simulink library "uavsimblockset"  (Simulink 8.6)
settings: Solver=ode45  StartTime=0.0  StopTime=10.0  RelTol=1e-3
undefined symbols (not defined in the file or in its folder): aircraftmask_displayVortices, aircraftmask_ID, DiscIntNeverNeededParam, uavsim
undefined symbols (not defined in the file): aircraftmask_originNED_ECEF_rrm, aircraftmask_p0_NED_m, aircraftmask_phithetapsi0, aircraftmask_pqr0, aircraftmask_uvw0, fflib_degdegm2rrm, flat2lla
libraries: uavsimBlockset_ServoHS55 x5, aerolibtransform2 x4, aerolibutil x3, uavsimBlockset_UAV3DInterface x3, uavsimblockset_SixDOFKinematics x2, simulink_extras x2, uavsimBlockset_Cularis_withUAV3D x2, uavsimBlockset_ElectricPropulsion x2, formationFlyingBlockset x2, uavsimBlockset_DerivedAerodynamicConditions x2, uavsimBlockset_alphabetaVa2uvw x1, uavsimBlockset_AirspeedController x1
(part 1 of 2)
settings Model: Creator=mstolle  LastModifiedBy=j.bolting

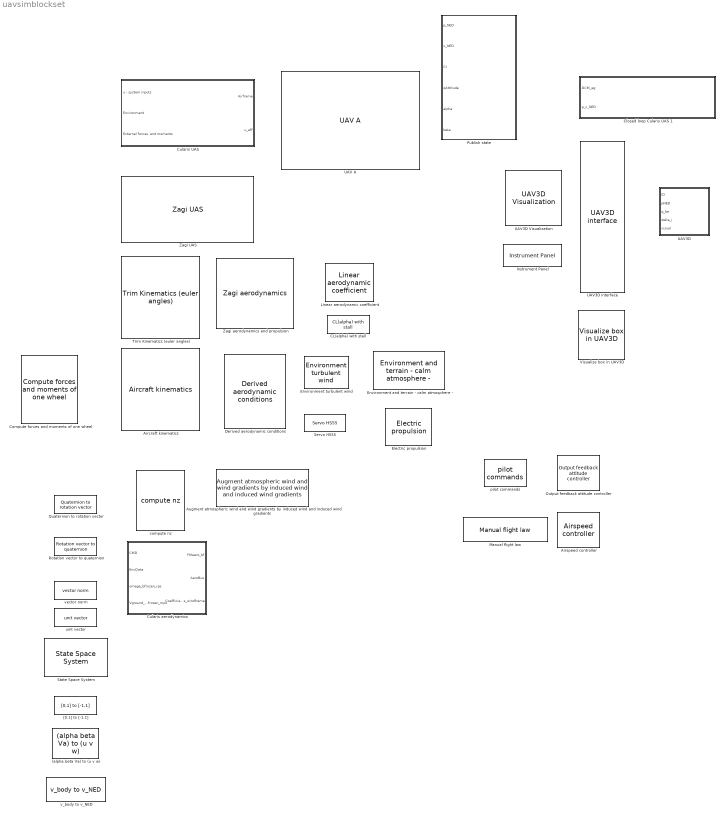
== system uavsimblockset ==
  (alpha beta Va) to (u v w) : uavsimBlockset_alphabetaVa2uvw/(alpha beta Va) to (u v w)
  Aircraft kinematics : uavsimblockset_SixDOFKinematics/Aircraft kinematics  mask_inertia="[ 0.98244, 0, -0.1204; 0,1.135,  0; -0.1204, 0,1.759]"  mask_mass=13.5  mask_P0_ECEF_rrm=mask_zagi_p0_ECEF_lla  mask_originNED_ECEF_rrm=0  mask_uvw0=mask_aerosonde_uvw0  mask_phithetapsi0=mask_aerosonde_phithetapsi0  mask_omega0=mask_aerosonde_pqr0
  Airspeed controller : uavsimBlockset_AirspeedController/Airspeed controller  mask_K=0
  Augment atmospheric wind and wind gradients by induced wind and induced wind gradients : uavsimBlockset_AugmentWind/Augment atmospheric wind and wind gradients by induced wind and induced wind gradients
  CL(alpha) with stall : uavsimBlockset_LiftCoefficientWithStall/CL(alpha) with stall  mask_M=0  mask_alpha0=0  mask_CL_0=0  mask_CL_alpha=0
  Closed loop Cularis UAS 1 : Subsystem  mask{closedloopmask_ID=2}
      mask prompts: closedloopmask_ID "UAS ID"
  Compute forces and moments of one wheel : uavsimBlockset_landinggear_onwheel/Compute forces and moments of one wheel
  Cularis UAS : Subsystem  mask{mask_cularis_phithetapsi0=aircraftmask_phithetapsi0, mask_cularis_p0_ECEF_lla=fflib_degdegm2rrm(flat2lla(aircraftmask_p0_NED_m, rad2deg(aircraftmask_originNED_ECEF_rrm(1:2)), 0, aircraftmask_originNED_ECEF_rrm(3))), mask_cularis_originNED_ECEF_rrm=aircraftmask_originNED_ECEF_rrm, mask_cularis_pqr0=aircraftmask_pqr0, mask_cularis_uvw0=aircraftmask_uvw0, uavsim=uavsim}
      mask prompts: mask_cularis_phithetapsi0 "Initial euler angles [rad]"; mask_cularis_p0_ECEF_lla "Initial position ECEF [rad rad m]"; mask_cularis_originNED_ECEF_rrm "Origin NED frame, ECEF-WGS84, [rad rad m]"; mask_cularis_pqr0 "Initial body rotation rates [rad/s]"; mask_cularis_uvw0 "Initial velocity body frame [m/s]"; uavsim "Parameter set"
      mask Display: image(imread('images/cularis.png'),[.3, .3, .4, .4])
  Cularis aerodynamics : Subsystem  AncestorBlock=uavsimBlockset_Cularis_Aerandpropulsion/Cularis aerodynamics and propulsion
  Derived aerodynamic conditions : uavsimBlockset_DerivedAerodynamicConditions/Derived aerodynamic conditions
  Electric propulsion : uavsimBlockset_ElectricPropulsion/Electric propulsion  mask_C_prop=0  mask_S_prop=0  mask_k_motor=0
  Environment turbulent wind : uavsimBlockset_Environment_turbulentWind/Environment turbulent wind  mask_constantwind_NED_mps=[0 0 0]'  mask_wingspan=1  mask_windON=mask_windON  mask_turbulenceON=1
  Environment and terrain - calm atmosphere - : uavsimBlockset_Environment_calmAtmosphere/Environment and terrain - calm atmosphere -  SystemSampleTime=-1
  Instrument Panel : uavsimBlockset_InstrumentPanel/Instrument Panel
  Linear aerodynamic coefficient : uavsimBlockset_LinearAerodynamicCoefficient/Linear aerodynamic coefficient  mask_C_0=0  mask_C_alpha=0  mask_C_beta=0  mask_C_alphaDot=0  mask_C_betaDot=0  mask_C_p=0  mask_C_q=0  mask_C_r=0  mask_C_delta_a=0  mask_C_delta_e=0  mask_C_delta_r=0  mask_C_delta_f=0  mask_C_Mach=0
  Manual flight law : uavsimBlockset_ManualLaw/Manual flight law  mask_scale_da=0  mask_scale_de=0  mask_scale_dr=0  mask_scale_den=0  mask_scale_df=0  mask_utrim=0
  Output feedback attitude controller : uavsimBlockset_quaternionAttitudeController/Output feedback attitude controller  mask_K=uavsim.control.linear.K_attitude
  Publish state : Subsystem  mask{mask_ID=aircraftmask_ID}
      mask prompts: mask_ID "ID"
  Quaternion to rotation vector : uavsimBlockset_Quaternion2Rotationvector/Quaternion to rotation vector
  Rotation vector to quaternion : uavsimBlockset_RotationVector2Quaternion/Rotation vector to quaternion
  Servo HS55 : uavsimBlockset_ServoHS55/Servo HS55  deflectionLimits_rad=[deg2rad(-45) deg2rad(45)]  rateLimit_enabled=on  outputLimit_enabled=on  mask_initialPosition=0
  State Space System : uavsimBlockset_StateSpaceSystem/State Space System  mask_a=0  mask_b=0  mask_c=0  mask_d=0  mask_x0=0
  Trim Kinematics (euler angles) : uavsimblockset_TrimKinematics/Trim Kinematics (euler angles)  mask_inertia=0  mask_mass=0  mask_P0_ECEF_m=0  mask_uvw0=0  mask_phithetapsi0=0  mask_omega0=0
  UAV A : uavsimBlockset_Cularis_withUAV3D/UAV A  aircraftmask_phithetapsi0=[uavsim.cularis.phithetapsi0(1:2); deg2rad(-30)]'  aircraftmask_p0_NED_m=[0 0 -50]  aircraftmask_originNED_ECEF_rrm=uavsim.originNED_ECEF_radradm  aircraftmask_pqr0=uavsim.cularis.omega0  aircraftmask_uvw0=uavsim.cularis.uvw0  aircraftmask_phithetapsi_trim=uavsim.cularis.phithetapsi0  aircraftmask_ID=1  aircraftmask_wakevortexenabled=off  aircraftmask_navigationLaw=4  uavsim=uavsim  leaderID=0  aircraftmask_displayUAV3D=on  aircraftmask_displayVortices=off
  UAV3D : Subsystem
  UAV3D Visualization : uavsimBlockset_UAV3DVisualization/UAV3D Visualization  mask_visual=0
  UAV3D interface : uavsimBlockset_UAV3DInterface/UAV3D interface  ip='localhost'  udpport=4445
  Visualize box in UAV3D : uavsimBlockset_UAV3D_visualizeBox/Visualize box in UAV3D
  Zagi UAS : uavsimBlockset_ZagiUAS/Zagi UAS  mask_zagi_phithetapsi0=[0 0 0]'  mask_zagi_p0_ECEF_lla=[0 0 50]'  mask_zagi_originNED_ECEF_rrm=0  mask_zagi_pqr0=[0 0 0]'  mask_zagi_uvw0=[30 0 0]  uavsim=uavsim
  Zagi aerodynamics and propulsion : uavsimBlockset_Zagi_Aerandpropulsion/Zagi aerodynamics
  "[0,1] to [-1,1]" : uavsimBlockset_01to11/[0,1] to [-1,1]
  compute nz : uavsimBlockset_ComputeNz/compute nz
  pilot commands : uavsimblockset_PilotCommands/pilot commands
  unit vector : uavsimBlockset_UnitVector/unit vector
  v_body to v_NED : uavsimblockset_vbody2vNED/v_body to v_NED
  vector norm : uavsimBlockset_VectorNorm/vector norm

== system uavsimblockset/Closed loop Cularis UAS 1 ==
  DCM_eg : Inport
  p_c_NED : Inport  Port=2
  Controllers : Subsystem
  UAV : uavsimBlockset_Cularis_withUAV3D/UAV A  aircraftmask_phithetapsi0=uavsim.formation(closedloopmask_ID).phithetapsi0  aircraftmask_p0_NED_m=uavsim.formation(closedloopmask_ID).p0_NED'  aircraftmask_originNED_ECEF_rrm=uavsim.originNED_ECEF_radradm  aircraftmask_pqr0=uavsim.formation(closedloopmask_ID).omega0  aircraftmask_uvw0=uavsim.formation(closedloopmask_ID).uvw0  aircraftmask_phithetapsi_trim=uavsim.formation(closedloopmask_ID).phithetapsi0  aircraftmask_ID=closedloopmask_ID  aircraftmask_wakevortexenabled=off  aircraftmask_navigationLaw=-1  uavsim=uavsim  leaderID=0  aircraftmask_displayUAV3D=on  aircraftmask_displayVortices=off
  wires:
  Controllers/1(u) -> UAV/1  "u_c"
  p_c_NED/1 -> Controllers/4(p_c_NED)
  DCM_eg/1 -> Controllers/3(DCM_eg)
  UAV/2 -> Controllers/2(id)
  UAV/1 -> Controllers/1(AirframeBus)

== system uavsimblockset/Cularis UAS ==
  u - system inputs : Inport  OutDataTypeStr=Bus: CMD
  Environment : Inport  Port=2  OutDataTypeStr=Bus: Environment
  External forces  and moments : Inport  Port=3
  Actuator dynamics neglected? : ManualSwitch  CurrentSetting=0
  Cularis actuators - time behaviour : Subsystem  TreatAsAtomicUnit=on
  ID2 : Constant  Value=aircraftmask_displayVortices
  Nonlinear aircraft model : Subsystem
  Publish state : Subsystem  TreatAsAtomicUnit=on
  Terminator1 : Terminator
  Wake vortex effects : formationFlyingBlockset/Wake vortex effects
  Airframe : Outport  OutDataTypeStr=Bus: Airframe
  u_eff : Outport  Port=2  OutDataTypeStr=Bus: CMD
  wires:
  u - system inputs/1 -> Cularis actuators - time behaviour/1(computed inputs), Actuator dynamics neglected?/2
  Cularis actuators - time behaviour/1(Effective  plant inputs) -> Actuator dynamics neglected?/1
  ID2/1 -> Wake vortex effects/4
  Publish state/2(Ci_w_out) -> Wake vortex effects/3
  Publish state/1(AiframeBus_out) -> Wake vortex effects/1
  Wake vortex effects/1 -> Nonlinear aircraft model/2(EnvData)
  Environment/1 -> Wake vortex effects/2
  Nonlinear aircraft model/3(FMprop) -> Terminator1/1
  Nonlinear aircraft model/2(Cwind) -> Publish state/2(Ci_w)
  Nonlinear aircraft model/1(Airframe) -> Airframe/1, Publish state/1(AirframeBus)
  Actuator dynamics neglected?/1 -> u_eff/1, Nonlinear aircraft model/1(CMD)
  External forces  and moments/1 -> Nonlinear aircraft model/3(FM_external)

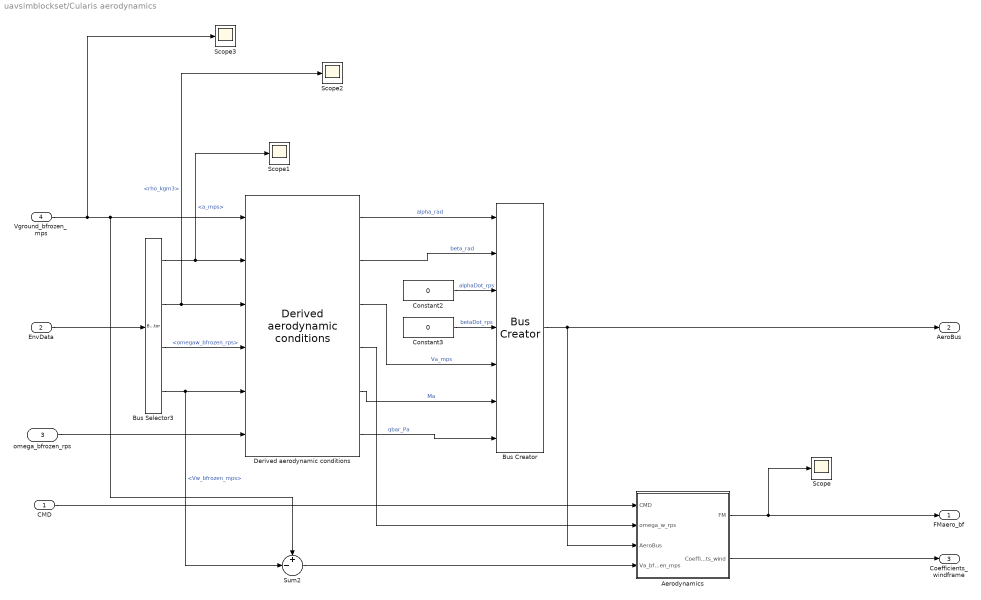
== system uavsimblockset/Cularis aerodynamics ==
  CMD : Inport  OutDataTypeStr=Bus: CMD
  EnvData : Inport  Port=2  OutDataTypeStr=Bus: Environment
  omega_bfrozen_rps : Inport  Port=3
  Vground_bfrozen_mps : Inport  Port=4
  Aerodynamics : Subsystem
  Bus Selector3 : BusSelector  OutputSignals=a_mps,rho_kgm3,omegaw_bfrozen_rps,Vw_bfrozen_mps
  Bus Creator : BusCreator  Inputs=7
  Constant2 : Constant  Value=0
  Constant3 : Constant  Value=0
  Derived aerodynamic conditions : uavsimBlockset_DerivedAerodynamicConditions/Derived aerodynamic conditions
  Scope{,1..3} (4 alike) : Scope
  Sum2 : Sum  Inputs=+-|  SaturateOnIntegerOverflow=on  InputSameDT=on  OutDataTypeStr=Inherit: Same as first input
  FMaero_bf : Outport
  AeroBus : Outport  Port=2  OutDataTypeStr=Bus: Aero
  Coefficients_windframe : Outport  Port=3
  wires:
  EnvData/1 -> Bus Selector3/1
  omega_bfrozen_rps/1 -> Derived aerodynamic conditions/6
  Aerodynamics/1(FM) -> FMaero_bf/1, Scope/1
  CMD/1 -> Aerodynamics/1(CMD)
  Aerodynamics/2(Coefficients_wind) -> Coefficients_windframe/1
  Bus Selector3/1 -> Derived aerodynamic conditions/2, Scope1/1  "<a_mps>"
  Bus Selector3/2 -> Derived aerodynamic conditions/3, Scope2/1  "<rho_kgm3>"
  Bus Selector3/3 -> Derived aerodynamic conditions/4  "<omegaw_bfrozen_rps>"
  Bus Selector3/4 -> Derived aerodynamic conditions/5, Sum2/2  "<Vw_bfrozen_mps>"
  Constant2/1 -> Bus Creator/3  "alphaDot_rps"
  Constant3/1 -> Bus Creator/4  "betaDot_rps"
  Vground_bfrozen_mps/1 -> Sum2/1, Derived aerodynamic conditions/1, Scope3/1
  Derived aerodynamic conditions/1 -> Bus Creator/1  "alpha_rad"
  Derived aerodynamic conditions/2 -> Bus Creator/2  "beta_rad"
  Derived aerodynamic conditions/3 -> Bus Creator/5  "Va_mps"
  Derived aerodynamic conditions/5 -> Bus Creator/6  "Ma"
  Derived aerodynamic conditions/6 -> Bus Creator/7  "qbar_Pa"
  Bus Creator/1 -> AeroBus/1, Aerodynamics/3(AeroBus)
  Sum2/1 -> Aerodynamics/4(Va_bfrozen_mps)
  Derived aerodynamic conditions/4 -> Aerodynamics/2(omega_w_rps)

== system uavsimblockset/Publish state ==
  p_NED : Inport
  v_NED : Inport  Port=2
  Cl : Inport  Port=3
  qAttitude : Inport  Port=4
  alpha : Inport  Port=5
  beta : Inport  Port=6
  Cularis vortex geometry parameters : formationFlyingBlockset/Cularis vortex geometry parameters  mask_ID=mask_ID
  Digital Clock : DigitalClock
  MATLAB Function1 : MATLAB Function  TreatAsAtomicUnit=on
  wires:
  Digital Clock/1 -> MATLAB Function1/8(tsim)
  Cularis vortex geometry parameters/1 -> MATLAB Function1/7(p)
  p_NED/1 -> MATLAB Function1/1(pNED)
  v_NED/1 -> MATLAB Function1/2(vNED)
  Cl/1 -> MATLAB Function1/3(CL)
  qAttitude/1 -> MATLAB Function1/4(qAttitude)
  alpha/1 -> MATLAB Function1/5(alpha)
  beta/1 -> MATLAB Function1/6(beta)

== system uavsimblockset/UAV3D ==
  ID : Inport
  pNED : Inport  Port=2
  q_be : Inport  Port=3
  delta_i : Inport  Port=4
  visual : Inport  Port=5
  Constant : Constant
  Demux : Demux  Outputs=5
  Demux1 : Demux
  Demux2 : Demux  Outputs=3
  UAV3D interface : uavsimBlockset_UAV3DInterface/UAV3D interface  ip='localhost'  udpport=4445
  wires:
  visual/1 -> UAV3D interface/14
  delta_i/1 -> Demux/1
  Demux/5 -> UAV3D interface/13
  Demux/4 -> UAV3D interface/12
  Demux/3 -> UAV3D interface/11
  Demux/2 -> UAV3D interface/10
  Demux/1 -> UAV3D interface/9
  Demux1/1 -> UAV3D interface/5
  Demux1/2 -> UAV3D interface/6
  Demux1/3 -> UAV3D interface/7
  Demux1/4 -> UAV3D interface/8
  q_be/1 -> Demux1/1
  Demux2/3 -> UAV3D interface/4
  Demux2/2 -> UAV3D interface/3
  Demux2/1 -> UAV3D interface/2
  pNED/1 -> Demux2/1
  ID/1 -> UAV3D interface/1
  Constant/1 -> UAV3D interface/Enable

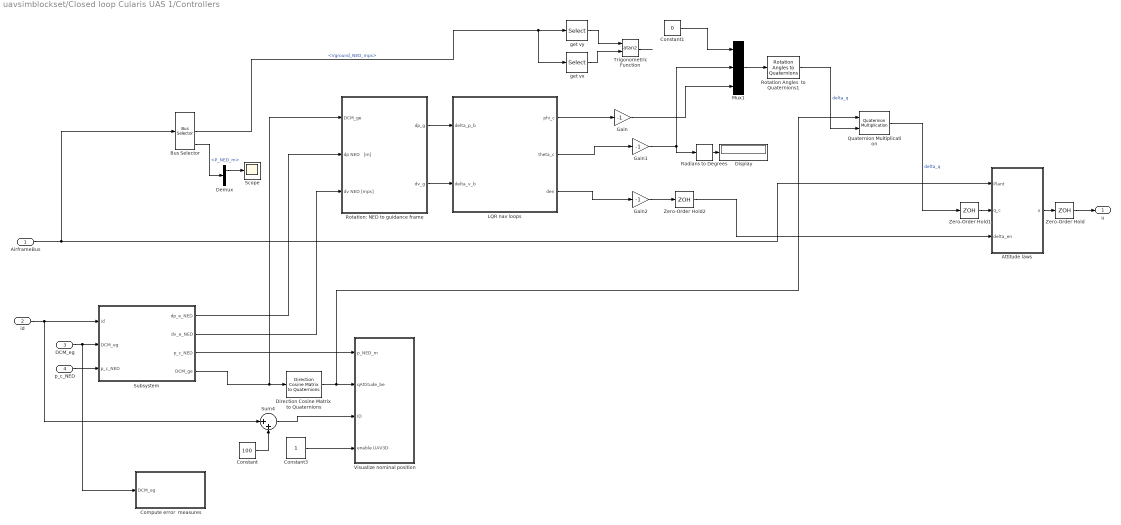
== system uavsimblockset/Closed loop Cularis UAS 1/Controllers ==
  AirframeBus : Inport
  id : Inport  Port=2
  DCM_eg : Inport  Port=3
  p_c_NED : Inport  Port=4
  Attitude laws : Subsystem  SystemSampleTime=uavsim.ap.hardware.dt_attitudeloops_s
  Bus Selector : BusSelector  OutputSignals=Kinematics.Attitude.DCM_be,Kinematics.Velocity.Vground_NED_mps,Kinematics.Position.P_NED_m
  Compute error  measures : Subsystem
  Constant : Constant  Value=100
  Constant1 : Constant  Value=0
  Constant3 : Constant
  Demux : Demux  Outputs=[2 1]
  Direction Cosine Matrix  to Quaternions : aerolibtransform2/Direction Cosine Matrix  to Quaternions
  Display : Display
  Gain : Gain  Gain=-1
  Gain1 : Gain  Gain=-1
  Gain2 : Gain  Gain=-1
  LQR nav loops : Subsystem  SystemSampleTime=uavsim.ap.hardware.dt_navigationloops_s
  Mux1 : Mux  Inputs=3
  Quaternion Multiplication : aerolibutil/Quaternion Multiplication
  Radians to Degrees : simulink_extras/Transformations/Radians to Degrees
  Rotation Angles  to Quaternions1 : aerolibtransform2/Rotation Angles to Quaternions  rotationOrder=ZYX
  Rotation: NED to guidance frame : Subsystem
  Scope : Scope
  Subsystem : Subsystem
  Sum4 : Sum  Inputs=|++
  Trigonometric Function : Trigonometry  Operator=atan2
  Visualize nominal position : Subsystem  TreatAsAtomicUnit=on  SystemSampleTime=uavsim.simConfig.tsample_UAV3D  mask{mask_3dmodel=1}
      mask prompts: mask_3dmodel "3D model"
      mask TypeOptions mask_3dmodel: 0 | 1 | 2 | 3
  Zero-Order Hold : ZeroOrderHold  SampleTime=uavsim.ap.tsampling_attitudelaws
  Zero-Order Hold1 : ZeroOrderHold  SampleTime=uavsim.ap.tsampling_guidancelaws
  Zero-Order Hold2 : ZeroOrderHold  SampleTime=uavsim.ap.tsampling_guidancelaws
  get vx : Selector  InputPortWidth=3  IndexOptions=Index vector (dialog)  Indices=[1]  OutputSizes=1
  get vy : Selector  InputPortWidth=3  IndexOptions=Index vector (dialog)  Indices=2  OutputSizes=1
  u : Outport
  wires:
  Rotation Angles  to Quaternions1/1 -> Quaternion Multiplication/2  "delta_q"
  Constant1/1 -> Mux1/1
  DCM_eg/1 -> Subsystem/2(DCM_eg), Compute error  measures/1(DCM_eg)
  Demux/1 -> Scope/1
  Bus Selector/3 -> Demux/1  "<P_NED_m>"
  Subsystem/2(dv_e_NED) -> Rotation: NED to guidance frame/3(dv NED [mps])
  Subsystem/1(dp_e_NED) -> Rotation: NED to guidance frame/2(dp NED   [m])
  Subsystem/4(DCM_ge) -> Direction Cosine Matrix  to Quaternions/1, Rotation: NED to guidance frame/1(DCM_ge)
  Subsystem/3("p_c_NED ") -> Visualize nominal position/1(p_NED_m)
  p_c_NED/1 -> Subsystem/3(p_c_NED)
  id/1 -> Subsystem/1(id), Sum4/1
  Zero-Order Hold2/1 -> Attitude laws/3(delta_en)
  Zero-Order Hold1/1 -> Attitude laws/2(q_c)
  Constant3/1 -> Visualize nominal position/4(enable UAV3D)
  Constant/1 -> Sum4/2
  Sum4/1 -> Visualize nominal position/3(ID)
  Direction Cosine Matrix  to Quaternions/1 -> Visualize nominal position/2(qAttitude_be), Quaternion Multiplication/1
  Bus Selector/2 -> get vy/1, get vx/1  "<Vground_NED_mps>"
  Radians to Degrees/1 -> Display/1
  Rotation: NED to guidance frame/1(dp_g) -> LQR nav loops/1(delta_p_b)
  Gain2/1 -> Zero-Order Hold2/1
  Rotation: NED to guidance frame/2(dv_g) -> LQR nav loops/2(delta_v_b)
  Quaternion Multiplication/1 -> Zero-Order Hold1/1  "delta_q"
  Attitude laws/1(u) -> Zero-Order Hold/1
  get vy/1 -> Trigonometric Function/1
  AirframeBus/1 -> Bus Selector/1, Attitude laws/1(Plant)
  get vx/1 -> Trigonometric Function/2
  Mux1/1 -> Rotation Angles  to Quaternions1/1
  Gain/1 -> Mux1/3
  Trigonometric Function/1 -> ?
  Gain1/1 -> Mux1/2, Radians to Degrees/1
  Zero-Order Hold/1 -> u/1
  LQR nav loops/1(phi_c) -> Gain/1
  LQR nav loops/2(theta_c) -> Gain1/1
  LQR nav loops/3(den) -> Gain2/1

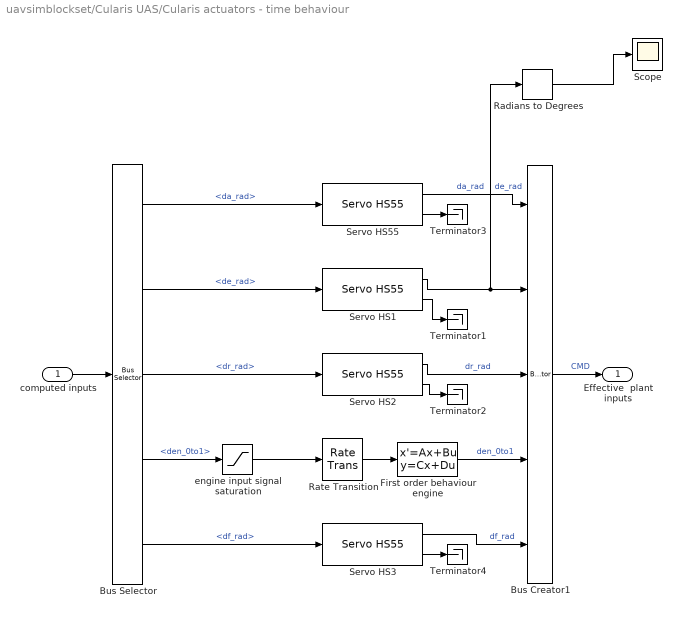
== system uavsimblockset/Cularis UAS/Cularis actuators - time behaviour ==
  computed inputs : Inport  OutDataTypeStr=Bus: CMD
  Bus Creator1 : BusCreator  Inputs=5  OutDataTypeStr=Bus: CMD  NonVirtualBus=on
  Bus Selector : BusSelector  OutputSignals=da_rad,de_rad,dr_rad,den_0to1,df_rad
  First order behaviour engine : StateSpace  A=-3.704  B=2  C=1.852  D=0  X0=uavsim.formation(aircraftmask_ID).u0.den/1.852
  Radians to Degrees : simulink_extras/Transformations/Radians to Degrees
  Rate Transition : RateTransition  Integrity=off
  Scope : Scope
  Servo HS1 : uavsimBlockset_ServoHS55/Servo HS55  deflectionLimits_rad=[deg2rad(-45) deg2rad(45)]  rateLimit_enabled=on  outputLimit_enabled=on  mask_initialPosition=uavsim.formation(aircraftmask_ID).u0.de
  Servo HS2 : uavsimBlockset_ServoHS55/Servo HS55  deflectionLimits_rad=[deg2rad(-45) deg2rad(45)]  rateLimit_enabled=on  outputLimit_enabled=on  mask_initialPosition=uavsim.formation(aircraftmask_ID).u0.dr
  Servo HS3 : uavsimBlockset_ServoHS55/Servo HS55  deflectionLimits_rad=[deg2rad(-10) deg2rad(90)]  rateLimit_enabled=on  outputLimit_enabled=on  mask_initialPosition=uavsim.formation(aircraftmask_ID).u0.df
  Servo HS55 : uavsimBlockset_ServoHS55/Servo HS55  deflectionLimits_rad=[deg2rad(-45) deg2rad(45)]  rateLimit_enabled=on  outputLimit_enabled=on  mask_initialPosition=uavsim.formation(aircraftmask_ID).u0.da
  Terminator{1..4} (4 alike) : Terminator
  engine input signal saturation : Saturate  UpperLimit=1  LowerLimit=0
  Effective  plant inputs : Outport  OutDataTypeStr=Bus: CMD
  wires:
  Radians to Degrees/1 -> Scope/1
  Servo HS55/2 -> Terminator3/1
  Servo HS1/2 -> Terminator1/1
  First order behaviour engine/1 -> Bus Creator1/4  "den_0to1"
  Servo HS3/2 -> Terminator4/1
  Servo HS2/2 -> Terminator2/1
  engine input signal saturation/1 -> Rate Transition/1
  Rate Transition/1 -> First order behaviour engine/1
  Bus Selector/1 -> Servo HS55/1  "<da_rad>"
  Servo HS55/1 -> Bus Creator1/1  "da_rad"
  Servo HS1/1 -> Bus Creator1/2, Radians to Degrees/1  "de_rad"
  Servo HS2/1 -> Bus Creator1/3  "dr_rad"
  Bus Selector/2 -> Servo HS1/1  "<de_rad>"
  Bus Selector/3 -> Servo HS2/1  "<dr_rad>"
  Bus Selector/4 -> engine input signal saturation/1  "<den_0to1>"
  computed inputs/1 -> Bus Selector/1
  Bus Creator1/1 -> Effective  plant inputs/1  "CMD"
  Bus Selector/5 -> Servo HS3/1  "<df_rad>"
  Servo HS3/1 -> Bus Creator1/5  "df_rad"

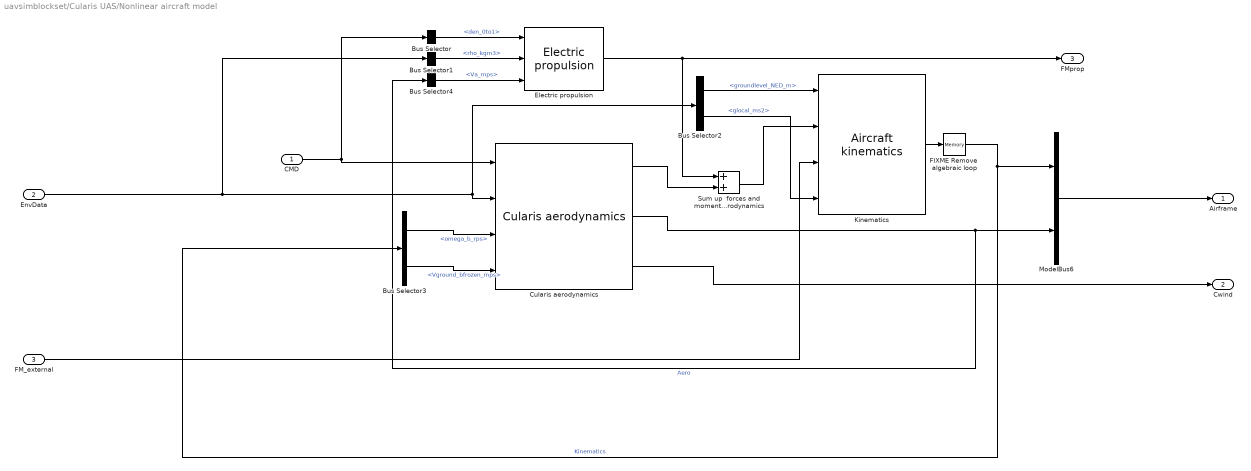
== system uavsimblockset/Cularis UAS/Nonlinear aircraft model ==
  CMD : Inport
  EnvData : Inport  Port=2
  FM_external : Inport  Port=3
  Bus Selector : BusSelector  OutputSignals=den_0to1
  Bus Selector1 : BusSelector  OutputSignals=rho_kgm3
  Bus Selector2 : BusSelector  OutputSignals=groundlevel_NED_m,glocal_ms2
  Bus Selector3 : BusSelector  OutputSignals=RotationalVelocity.omega_b_rps,Velocity.Vground_bfrozen_mps
  Bus Selector4 : BusSelector  OutputSignals=Va_mps
  Cularis aerodynamics : uavsimBlockset_Cularis_Aerandpropulsion/Cularis aerodynamics  SystemSampleTime=-1
  Electric propulsion : uavsimBlockset_ElectricPropulsion/Electric propulsion  mask_C_prop=uavsim.cularis.C_prop  mask_S_prop=uavsim.cularis.S_prop  mask_k_motor=uavsim.cularis.k_motor
  FIXME Remove  algebraic loop : Memory  X0=1e-6
  Kinematics : uavsimblockset_SixDOFKinematics/Aircraft kinematics  mask_inertia=uavsim.cularis.inertiaTensor  mask_mass=uavsim.cularis.mass  mask_P0_ECEF_rrm=mask_cularis_p0_ECEF_lla  mask_originNED_ECEF_rrm=mask_cularis_originNED_ECEF_rrm  mask_uvw0=mask_cularis_uvw0  mask_phithetapsi0=mask_cularis_phithetapsi0  mask_omega0=mask_cularis_pqr0
  ModelBus6 : BusCreator  Inputs=2  OutDataTypeStr=Bus: Airframe  NonVirtualBus=on
  Sum up  forces and moments of engine and aircraft aerodynamics : Sum
  Airframe : Outport  OutDataTypeStr=Bus: Airframe
  Cwind : Outport  Port=2
  FMprop : Outport  Port=3
  wires:
  Electric propulsion/1 -> FMprop/1, Sum up  forces and moments of engine and aircraft aerodynamics/1
  CMD/1 -> Bus Selector/1, Cularis aerodynamics/1
  Bus Selector/1 -> Electric propulsion/1  "<den_0to1>"
  Bus Selector1/1 -> Electric propulsion/2  "<rho_kgm3>"
  Bus Selector4/1 -> Electric propulsion/3  "<Va_mps>"
  Kinematics/1 -> FIXME Remove  algebraic loop/1
  Sum up  forces and moments of engine and aircraft aerodynamics/1 -> Kinematics/2
  Cularis aerodynamics/1 -> Sum up  forces and moments of engine and aircraft aerodynamics/2
  Cularis aerodynamics/3 -> Cwind/1
  FM_external/1 -> Kinematics/3
  EnvData/1 -> Bus Selector2/1, Cularis aerodynamics/2, Bus Selector1/1
  Cularis aerodynamics/2 -> ModelBus6/2, Bus Selector4/1  "Aero"
  ModelBus6/1 -> Airframe/1
  Bus Selector3/2 -> Cularis aerodynamics/4  "<Vground_bfrozen_mps>"
  Bus Selector3/1 -> Cularis aerodynamics/3  "<omega_b_rps>"
  Bus Selector2/2 -> Kinematics/4  "<glocal_ms2>"
  Bus Selector2/1 -> Kinematics/1  "<groundlevel_NED_m>"
  FIXME Remove  algebraic loop/1 -> Bus Selector3/1, ModelBus6/1  "Kinematics"

== system uavsimblockset/Cularis UAS/Publish state ==
  AirframeBus : Inport  OutDataTypeStr=Bus: Airframe
  Ci_w : Inport  Port=2
  Subsystem : Subsystem
  AiframeBus_out : Outport  OutDataTypeStr=Bus: Airframe
  Ci_w_out : Outport  Port=2
  wires:
  Ci_w/1 -> Subsystem/2(Ci_w), Ci_w_out/1
  AirframeBus/1 -> Subsystem/1(AirframeBus), AiframeBus_out/1

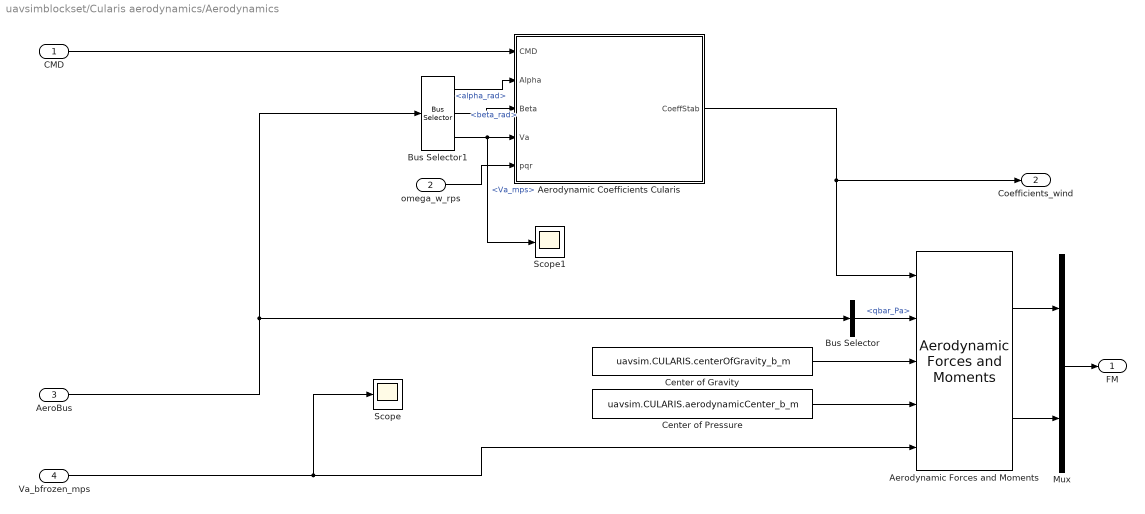
== system uavsimblockset/Cularis aerodynamics/Aerodynamics ==
  CMD : Inport  OutDataTypeStr=Bus: CMD
  omega_w_rps : Inport  Port=2
  AeroBus : Inport  Port=3  OutDataTypeStr=Bus: Aero
  Va_bfrozen_mps : Inport  Port=4
  Aerodynamic Coefficients Cularis : Subsystem
  "Aerodynamic Forces and Moments " : aerolibadyn/Aerodynamic Forces and Moments   inputAxes=Wind  outputForceAxes=Body  outputMomentAxes=Body  S=uavsim.CULARIS.S  b=uavsim.CULARIS.b  cbar=uavsim.CULARIS.c
  Bus Selector1 : BusSelector  OutputSignals=alpha_rad,beta_rad,Va_mps
  Bus Selector : BusSelector  OutputSignals=qbar_Pa
  Center of Gravity : Constant  Value=uavsim.CULARIS.centerOfGravity_b_m  SampleTime=0
  Center of Pressure : Constant  Value=uavsim.CULARIS.aerodynamicCenter_b_m  SampleTime=0
  Mux : Mux  Inputs=2
  Scope : Scope
  Scope1 : Scope
  FM : Outport
  Coefficients_wind : Outport  Port=2
  wires:
  "Aerodynamic Forces and Moments "/2 -> Mux/2
  Aerodynamic Coefficients Cularis/1(CoeffStab) -> "Aerodynamic Forces and Moments "/1, Coefficients_wind/1
  "Aerodynamic Forces and Moments "/1 -> Mux/1
  Center of Gravity/1 -> "Aerodynamic Forces and Moments "/3
  Center of Pressure/1 -> "Aerodynamic Forces and Moments "/4
  CMD/1 -> Aerodynamic Coefficients Cularis/1(CMD)
  Mux/1 -> FM/1
  Bus Selector/1 -> "Aerodynamic Forces and Moments "/2  "<qbar_Pa>"
  AeroBus/1 -> Bus Selector/1, Bus Selector1/1
  Bus Selector1/1 -> Aerodynamic Coefficients Cularis/2(Alpha)  "<alpha_rad>"
  Bus Selector1/2 -> Aerodynamic Coefficients Cularis/3(Beta)  "<beta_rad>"
  Bus Selector1/3 -> Aerodynamic Coefficients Cularis/4(Va), Scope1/1  "<Va_mps>"
  omega_w_rps/1 -> Aerodynamic Coefficients Cularis/5(pqr)
  Va_bfrozen_mps/1 -> "Aerodynamic Forces and Moments "/5, Scope/1

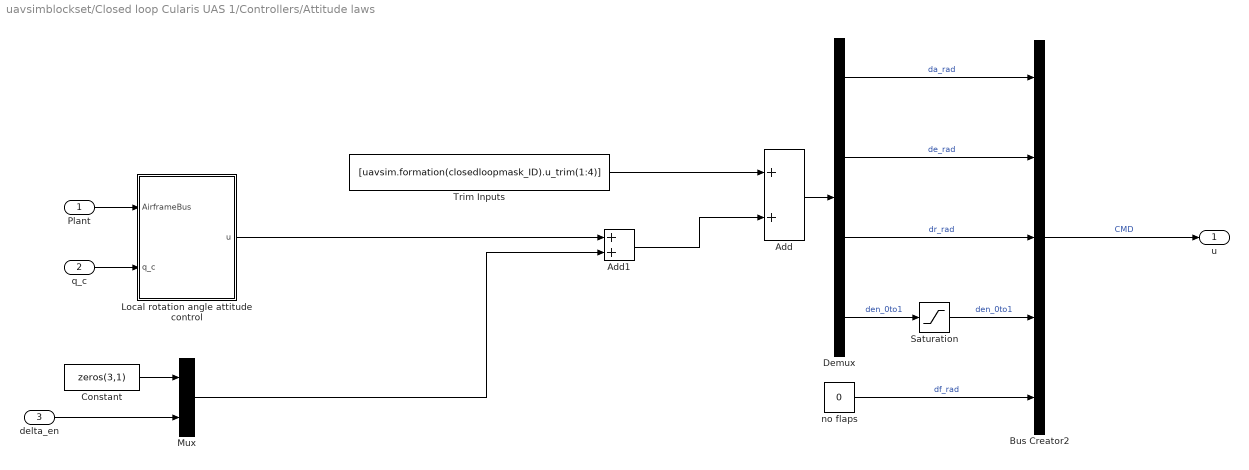
== system uavsimblockset/Closed loop Cularis UAS 1/Controllers/Attitude laws ==
  Plant : Inport  OutDataTypeStr=Bus: Airframe
  q_c : Inport  Port=2
  delta_en : Inport  Port=3
  Add : Sum
  Add1 : Sum
  Bus Creator2 : BusCreator  Inputs=5  OutDataTypeStr=Bus: CMD  NonVirtualBus=on
  Constant : Constant  Value=zeros(3,1)
  Demux : Demux
  Local rotation angle attitude  control : Subsystem
  Mux : Mux  Inputs=2
  Saturation : Saturate  UpperLimit=1  LowerLimit=0
  Trim Inputs : Constant  Value=[uavsim.formation(closedloopmask_ID).u_trim(1:4)]
  no flaps : Constant  Value=0
  u : Outport  OutDataTypeStr=Bus: CMD
  wires:
  Demux/4 -> Saturation/1  "den_0to1"
  Local rotation angle attitude  control/1(u) -> Add1/1
  Bus Creator2/1 -> u/1  "CMD"
  Demux/3 -> Bus Creator2/3  "dr_rad"
  Saturation/1 -> Bus Creator2/4  "den_0to1"
  Demux/1 -> Bus Creator2/1  "da_rad"
  Demux/2 -> Bus Creator2/2  "de_rad"
  Trim Inputs/1 -> Add/1
  Add/1 -> Demux/1
  Plant/1 -> Local rotation angle attitude  control/1(AirframeBus)
  q_c/1 -> Local rotation angle attitude  control/2(q_c)
  Constant/1 -> Mux/1
  Mux/1 -> Add1/2
  Add1/1 -> Add/2
  delta_en/1 -> Mux/2
  no flaps/1 -> Bus Creator2/5  "df_rad"

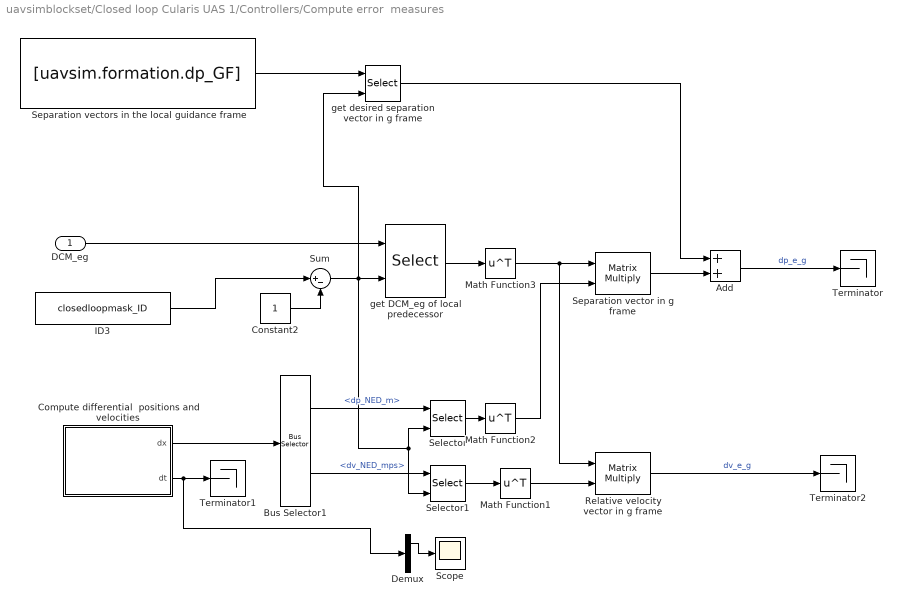
== system uavsimblockset/Closed loop Cularis UAS 1/Controllers/Compute error  measures ==
  DCM_eg : Inport
  Add : Sum
  Bus Selector1 : BusSelector  OutputSignals=dp_NED_m,dv_NED_mps
  Compute differential  positions and velocities : MATLAB Function  TreatAsAtomicUnit=on
  Constant2 : Constant
  Demux : Demux  Outputs=[4 6]
  ID3 : Constant  Value=closedloopmask_ID
  Math Function1 : Math  Operator=transpose  SaturateOnIntegerOverflow=on
  Math Function2 : Math  Operator=transpose  SaturateOnIntegerOverflow=on
  Math Function3 : Math  Operator=transpose  SaturateOnIntegerOverflow=on
  Relative velocity vector in g frame : Product  Multiplication=Matrix(*)
  Scope : Scope
  Selector : Selector  NumberOfDimensions=2  InputPortWidth=3  IndexOptions=Index vector (port),Select all  Indices=1,1:3  OutputSizes=1,1
  Selector1 : Selector  NumberOfDimensions=2  InputPortWidth=3  IndexOptions=Index vector (port),Index vector (dialog)  Indices=1,1:3  OutputSizes=1,1
  Separation vector in g frame : Product  Multiplication=Matrix(*)
  Separation vectors in the local guidance frame : Constant  Value=[uavsim.formation.dp_GF]
  Sum : Sum  Inputs=|+-
  Terminator : Terminator
  Terminator1 : Terminator
  Terminator2 : Terminator
  get DCM_eg of local predecessor : Selector  NumberOfDimensions=3  InputPortWidth=3  IndexOptions=Index vector (dialog),Index vector (dialog),Index vector (port)  Indices=1:3,1:3,1  OutputSizes=1,1,1
  get desired separation vector in g frame : Selector  NumberOfDimensions=2  InputPortWidth=3  IndexOptions=Select all,Index vector (port)  Indices=1,1:3  OutputSizes=1,1
  wires:
  Demux/1 -> Scope/1
  get desired separation vector in g frame/1 -> Add/1
  Compute differential  positions and velocities/2(dt) -> Terminator1/1, Demux/1
  Math Function3/1 -> Separation vector in g frame/1, Relative velocity vector in g frame/1
  Math Function1/1 -> Relative velocity vector in g frame/2
  Relative velocity vector in g frame/1 -> Terminator2/1  "dv_e_g"
  Add/1 -> Terminator/1  "dp_e_g"
  Separation vector in g frame/1 -> Add/2
  Selector1/1 -> Math Function1/1
  Math Function2/1 -> Separation vector in g frame/2
  get DCM_eg of local predecessor/1 -> Math Function3/1
  Sum/1 -> get DCM_eg of local predecessor/2, Selector/2, Selector1/2, get desired separation vector in g frame/2
  ID3/1 -> Sum/1
  Selector/1 -> Math Function2/1
  Compute differential  positions and velocities/1(dx) -> Bus Selector1/1
  Bus Selector1/2 -> Selector1/1  "<dv_NED_mps>"
  Bus Selector1/1 -> Selector/1  "<dp_NED_m>"
  Constant2/1 -> Sum/2
  DCM_eg/1 -> get DCM_eg of local predecessor/1
  Separation vectors in the local guidance frame/1 -> get desired separation vector in g frame/1

== system uavsimblockset/Closed loop Cularis UAS 1/Controllers/LQR nav loops ==
  delta_p_b : Inport
  delta_v_b : Inport  Port=2
  C nav lateral : Subsystem
  C nav longi : Subsystem
  get vz VLF : Selector  InputPortWidth=3  IndexOptions=Index vector (dialog)  Indices=3  OutputSizes=1
  get vz VLF1 : Selector  InputPortWidth=3  IndexOptions=Index vector (dialog)  Indices=1  OutputSizes=1
  get x VLF : Selector  InputPortWidth=3  IndexOptions=Index vector (dialog)  Indices=1  OutputSizes=1
  get z VLF : Selector  InputPortWidth=3  IndexOptions=Index vector (dialog)  Indices=3  OutputSizes=1
  phi_c : Outport  PortDimensions=1
  theta_c : Outport  Port=2  PortDimensions=1
  den : Outport  Port=3  PortDimensions=1
  wires:
  get vz VLF1/1 -> C nav longi/1(dvx)
  get vz VLF/1 -> C nav longi/2(dvz)
  get x VLF/1 -> C nav longi/3(dx)
  get z VLF/1 -> C nav longi/4(dz)
  C nav lateral/1(phi_c) -> phi_c/1
  delta_v_b/1 -> get vz VLF/1, get vz VLF1/1, C nav lateral/2(v_LTF)
  delta_p_b/1 -> get z VLF/1, get x VLF/1, C nav lateral/1(p_LTF)
  C nav longi/1(theta_c) -> theta_c/1
  C nav longi/2(den) -> den/1

== system uavsimblockset/Closed loop Cularis UAS 1/Controllers/Rotation: NED to guidance frame ==
  DCM_ge : Inport
  dp NED   [m] : Inport  Port=2
  dv NED [mps] : Inport  Port=3
  Rotate position vector from NED to LS frame : Product  Multiplication=Matrix(*)
  Rotate velocity vector from NED to LS frame : Product  Multiplication=Matrix(*)
  dp_g : Outport
  dv_g : Outport  Port=2
  wires:
  DCM_ge/1 -> Rotate position vector from NED to LS frame/1, Rotate velocity vector from NED to LS frame/1
  dv NED [mps]/1 -> Rotate velocity vector from NED to LS frame/2
  dp NED   [m]/1 -> Rotate position vector from NED to LS frame/2
  Rotate position vector from NED to LS frame/1 -> dp_g/1
  Rotate velocity vector from NED to LS frame/1 -> dv_g/1

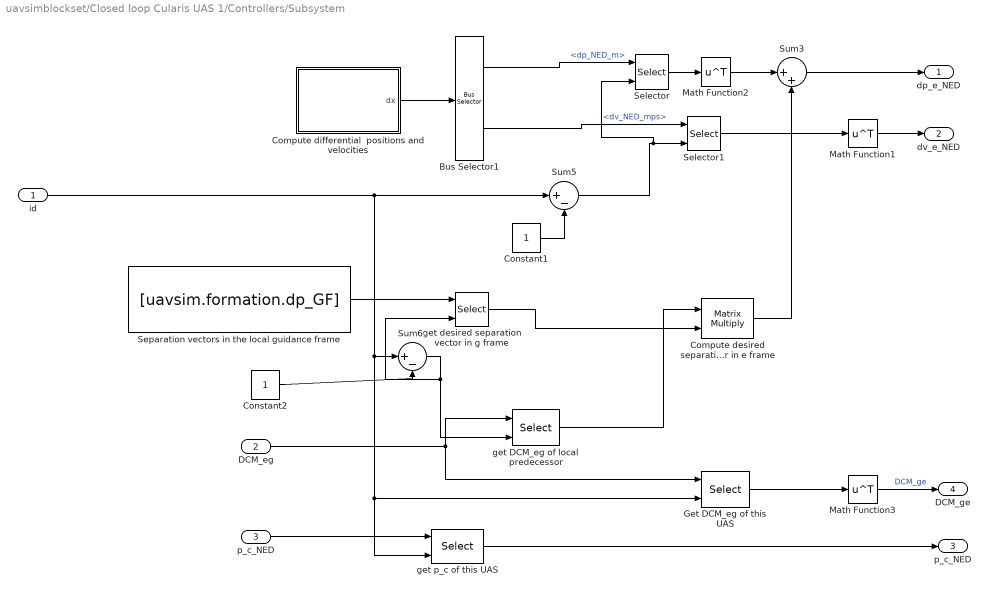
== system uavsimblockset/Closed loop Cularis UAS 1/Controllers/Subsystem ==
  id : Inport
  DCM_eg : Inport  Port=2
  p_c_NED : Inport  Port=3
  Bus Selector1 : BusSelector  OutputSignals=dp_NED_m,dv_NED_mps
  Compute desired separation vector in e frame : Product  Multiplication=Matrix(*)
  Compute differential  positions and velocities : MATLAB Function  TreatAsAtomicUnit=on
  Constant1 : Constant
  Constant2 : Constant
  Get DCM_eg of this UAS : Selector  NumberOfDimensions=3  InputPortWidth=3  IndexOptions=Index vector (dialog),Index vector (dialog),Index vector (port)  Indices=1:3,1:3,1  OutputSizes=1,1,1
  Math Function1 : Math  Operator=transpose  SaturateOnIntegerOverflow=on
  Math Function2 : Math  Operator=transpose  SaturateOnIntegerOverflow=on
  Math Function3 : Math  Operator=transpose  SaturateOnIntegerOverflow=on
  Selector : Selector  NumberOfDimensions=2  InputPortWidth=3  IndexOptions=Index vector (port),Select all  Indices=1,1:3  OutputSizes=1,1
  Selector1 : Selector  NumberOfDimensions=2  InputPortWidth=3  IndexOptions=Index vector (port),Index vector (dialog)  Indices=1,1:3  OutputSizes=1,1
  Separation vectors in the local guidance frame : Constant  Value=[uavsim.formation.dp_GF]
  Sum3 : Sum  Inputs=|++
  Sum5 : Sum  Inputs=|+-
  Sum6 : Sum  Inputs=|+-
  get DCM_eg of local predecessor : Selector  NumberOfDimensions=3  InputPortWidth=3  IndexOptions=Index vector (dialog),Index vector (dialog),Index vector (port)  Indices=1:3,1:3,1  OutputSizes=1,1,1
  get desired separation vector in g frame : Selector  NumberOfDimensions=2  InputPortWidth=3  IndexOptions=Select all,Index vector (port)  Indices=1,1:3  OutputSizes=1,1
  get p_c of this UAS : Selector  NumberOfDimensions=2  InputPortWidth=3  IndexOptions=Select all,Index vector (port)  Indices=1,1:3  OutputSizes=1,1
  dp_e_NED : Outport
  dv_e_NED : Outport  Port=2
  "p_c_NED " : Outport  Port=3
  DCM_ge : Outport  Port=4
  wires:
  id/1 -> Sum5/1, Get DCM_eg of this UAS/2, get p_c of this UAS/2, Sum6/1
  Compute desired separation vector in e frame/1 -> Sum3/2
  Math Function2/1 -> Sum3/1
  get desired separation vector in g frame/1 -> Compute desired separation vector in e frame/2
  Get DCM_eg of this UAS/1 -> Math Function3/1
  Separation vectors in the local guidance frame/1 -> get desired separation vector in g frame/1
  DCM_eg/1 -> Get DCM_eg of this UAS/1, get DCM_eg of local predecessor/1
  Selector/1 -> Math Function2/1
  Sum6/1 -> get desired separation vector in g frame/2, get DCM_eg of local predecessor/2
  Constant2/1 -> Sum6/2
  get DCM_eg of local predecessor/1 -> Compute desired separation vector in e frame/1
  Bus Selector1/1 -> Selector/1  "<dp_NED_m>"
  Bus Selector1/2 -> Selector1/1  "<dv_NED_mps>"
  Selector1/1 -> Math Function1/1
  Compute differential  positions and velocities/1(dx) -> Bus Selector1/1
  Sum5/1 -> Selector1/2, Selector/2
  Math Function3/1 -> DCM_ge/1  "DCM_ge"
  Constant1/1 -> Sum5/2
  get p_c of this UAS/1 -> "p_c_NED "/1
  p_c_NED/1 -> get p_c of this UAS/1
  Math Function1/1 -> dv_e_NED/1
  Sum3/1 -> dp_e_NED/1

== system uavsimblockset/Closed loop Cularis UAS 1/Controllers/Visualize nominal position ==
  p_NED_m : Inport
  qAttitude_be : Inport  Port=2
  ID : Inport  Port=3
  enable UAV3D : Inport  Port=4
  3D model : Constant  Value=mask_3dmodel
  Constant : Constant  Value=0
  Demux : Demux  Outputs=3
  Demux1 : Demux
  UAV3D interface : uavsimBlockset_UAV3DInterface/UAV3D interface  ip='localhost'  udpport=4445
  wires:
  enable UAV3D/1 -> UAV3D interface/Enable
  p_NED_m/1 -> Demux/1
  ID/1 -> UAV3D interface/1
  3D model/1 -> UAV3D interface/14
  Constant/1 -> UAV3D interface/9, UAV3D interface/10, UAV3D interface/11, UAV3D interface/12, UAV3D interface/13
  Demux1/3 -> UAV3D interface/7
  qAttitude_be/1 -> Demux1/1
  Demux1/4 -> UAV3D interface/8
  Demux1/2 -> UAV3D interface/6
  Demux1/1 -> UAV3D interface/5
  Demux/3 -> UAV3D interface/4
  Demux/2 -> UAV3D interface/3
  Demux/1 -> UAV3D interface/2

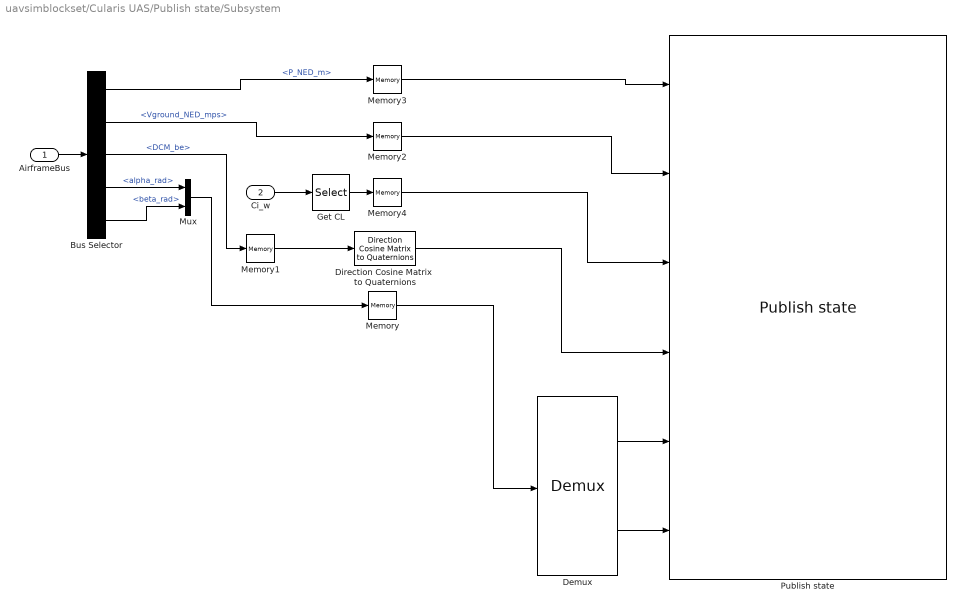
== system uavsimblockset/Cularis UAS/Publish state/Subsystem ==
  AirframeBus : Inport  OutDataTypeStr=Bus: Airframe
  Ci_w : Inport  Port=2
  Bus Selector : BusSelector  OutputSignals=Kinematics.Position.P_NED_m,Kinematics.Velocity.Vground_NED_mps,Kinematics.Attitude.DCM_be,Aero.alpha_rad,Aero.beta_rad
  Demux : Demux  Outputs=2
  Direction Cosine Matrix  to Quaternions : aerolibtransform2/Direction Cosine Matrix  to Quaternions
  Get CL : Selector  InputPortWidth=6  IndexOptions=Index vector (dialog)  Indices=3  OutputSizes=1
  Memory : Memory  X0=[0 0]
  Memory1 : Memory  X0=eye(3)
  Memory2 : Memory  X0=zeros(3,1)
  Memory3 : Memory  X0=zeros(3,1)
  Memory4 : Memory  X0=1
  Mux : Mux  Inputs=2
  Publish state : uavsimblockset/Publish state  mask_ID=aircraftmask_ID
  wires:
  Memory4/1 -> Publish state/3
  Memory3/1 -> Publish state/1
  Memory2/1 -> Publish state/2
  Memory1/1 -> Direction Cosine Matrix  to Quaternions/1
  Memory/1 -> Demux/1
  Mux/1 -> Memory/1
  Bus Selector/5 -> Mux/2  "<beta_rad>"
  Bus Selector/4 -> Mux/1  "<alpha_rad>"
  Bus Selector/3 -> Memory1/1  "<DCM_be>"
  Bus Selector/2 -> Memory2/1  "<Vground_NED_mps>"
  Bus Selector/1 -> Memory3/1  "<P_NED_m>"
  Direction Cosine Matrix  to Quaternions/1 -> Publish state/4
  Get CL/1 -> Memory4/1
  Ci_w/1 -> Get CL/1
  AirframeBus/1 -> Bus Selector/1
  Demux/2 -> Publish state/6
  Demux/1 -> Publish state/5

== system uavsimblockset/Cularis aerodynamics/Aerodynamics/Aerodynamic Coefficients Cularis ==
  CMD : Inport
  Alpha : Inport  Port=2
  Beta : Inport  Port=3
  Va : Inport  Port=4
  pqr : Inport  Port=5
  Actuator Increments : Subsystem
  Body rate damping Increments : Subsystem
  Datum Coefficients : Subsystem
  Sum1 : Sum  Inputs=+++  SaturateOnIntegerOverflow=on  InputSameDT=on  OutDataTypeStr=Inherit: Same as first input
  CoeffStab : Outport
  wires:
  Actuator Increments/1(CoeffAct) -> Sum1/2
  Body rate damping Increments/1(CoeffRate) -> Sum1/3
  Alpha/1 -> Datum Coefficients/1(Alpha)
  Va/1 -> Body rate damping Increments/2(Va)
  pqr/1 -> Body rate damping Increments/1(pqr)
  Beta/1 -> Datum Coefficients/2(Beta)
  CMD/1 -> Actuator Increments/1(CMD)
  Sum1/1 -> CoeffStab/1
  Datum Coefficients/1(CoeffDat) -> Sum1/1

== system uavsimblockset/Closed loop Cularis UAS 1/Controllers/Attitude laws/Local rotation angle attitude  control ==
  AirframeBus : Inport  OutDataTypeStr=Bus: Airframe
  q_c : Inport  Port=2
  Bus Selector : BusSelector  OutputSignals=Kinematics.RotationalVelocity.omega_b_rps
  "Compute local theta, phi, n_z" : Subsystem
  Constant : Constant  Value=[0 0]'
  Demux3 : Demux  Outputs=2
  Demux4 : Demux  Outputs=3
  Demux5 : Demux  Outputs=2
  Ground1 : Ground
  LQR pitch : Subsystem
  LQR roll : Subsystem
  Mux : Mux
  u : Outport
  wires:
  LQR roll/2(dr) -> Mux/3
  LQR roll/1(da) -> Mux/1
  LQR pitch/1(de) -> Mux/2
  Demux4/2 -> LQR pitch/1(q)
  Demux3/1 -> LQR pitch/2(theta)
  Demux5/1 -> LQR pitch/3(theta_c)
  Demux4/3 -> LQR roll/4(r)
  Demux4/1 -> LQR roll/3(p)
  Demux3/2 -> LQR roll/1(phi)
  Demux5/2 -> LQR roll/2(phi_c)
  "Compute local theta, phi, n_z"/1("theta, phi local") -> Demux3/1
  Bus Selector/1 -> Demux4/1  "<omega_b_rps>"
  Constant/1 -> Demux5/1
  Mux/1 -> u/1
  q_c/1 -> "Compute local theta, phi, n_z"/2(q_c)
  AirframeBus/1 -> Bus Selector/1, "Compute local theta, phi, n_z"/1(AirframeBus)
  Ground1/1 -> Mux/4

== system uavsimblockset/Closed loop Cularis UAS 1/Controllers/LQR nav loops/C nav lateral ==
  p_LTF : Inport
  v_LTF : Inport  Port=2
  Add : Sum  Inputs=+-
  Discrete-Time Integrator1 : DiscreteIntegrator  SampleTime=-1  ICPrevOutput=DiscIntNeverNeededParam  ICPrevScaledInput=DiscIntNeverNeededParam
  Ky : Gain  Gain=uavsim.ap.control.lquadr.latnav.K  Multiplication=Matrix(K*u)
  Mux1 : Mux  Inputs=3
  Selector : Selector  InputPortWidth=3  IndexOptions=Index vector (dialog)  Indices=2  OutputSizes=1
  Selector1 : Selector  InputPortWidth=3  IndexOptions=Index vector (dialog)  Indices=2  OutputSizes=1
  Step : Step  Time=12  After=0
  Trigonometric Function : Trigonometry  Operator=asin
  phi_c : Outport
  wires:
  Trigonometric Function/1 -> phi_c/1
  p_LTF/1 -> Selector/1
  v_LTF/1 -> Selector1/1
  Mux1/1 -> Ky/1
  Add/1 -> Discrete-Time Integrator1/1, Mux1/1
  Discrete-Time Integrator1/1 -> Mux1/3
  Selector1/1 -> Mux1/2
  Step/1 -> Add/2
  Selector/1 -> Add/1  "e"
  Ky/1 -> Trigonometric Function/1  "ny_c"

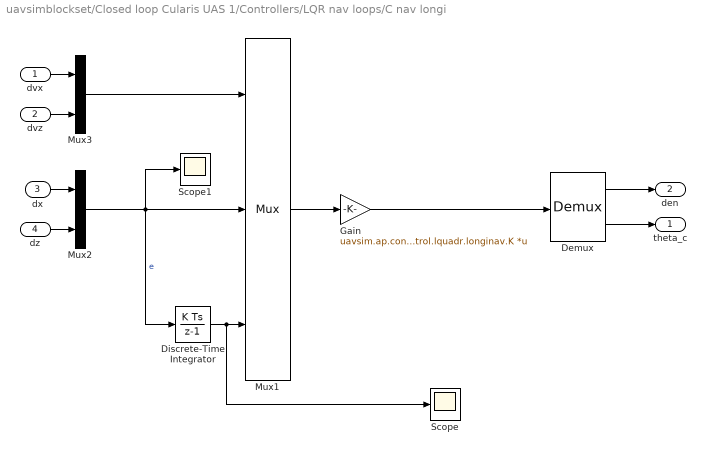
== system uavsimblockset/Closed loop Cularis UAS 1/Controllers/LQR nav loops/C nav longi ==
  dvx : Inport
  dvz : Inport  Port=2
  dx : Inport  Port=3
  dz : Inport  Port=4
  Demux : Demux  Outputs=2
  Discrete-Time Integrator : DiscreteIntegrator  gainval=1  InitialConditionSetting=State (most efficient)  SampleTime=-1  ICPrevOutput=DiscIntNeverNeededParam  ICPrevScaledInput=DiscIntNeverNeededParam
  Gain : Gain  Gain=uavsim.ap.control.lquadr.longinav.K  Multiplication=Matrix(K*u)
  Mux1 : Mux  Inputs=3
  Mux2 : Mux  Inputs=2
  Mux3 : Mux  Inputs=2
  Scope : Scope
  Scope1 : Scope
  theta_c : Outport
  den : Outport  Port=2
  wires:
  Mux3/1 -> Mux1/1
  dz/1 -> Mux2/2
  Gain/1 -> Demux/1
  Mux2/1 -> Mux1/2, Scope1/1, Discrete-Time Integrator/1  "e"
  Discrete-Time Integrator/1 -> Mux1/3, Scope/1
  dvx/1 -> Mux3/1
  dvz/1 -> Mux3/2
  dx/1 -> Mux2/1
  Demux/2 -> theta_c/1
  Demux/1 -> den/1
  Mux1/1 -> Gain/1

== system uavsimblockset/Cularis aerodynamics/Aerodynamics/Aerodynamic Coefficients Cularis/Actuator Increments ==
  CMD : Inport
  Aileron : Subsystem
  Bus Selector : BusSelector  OutputSignals=da_rad
  Bus Selector1 : BusSelector  OutputSignals=de_rad
  Bus Selector2 : BusSelector  OutputSignals=dr_rad
  Elevator : Subsystem
  Gain : Gain
  Gain1 : Gain
  Rudder : Subsystem
  Sum1 : Sum  Inputs=+++  SaturateOnIntegerOverflow=on  InputSameDT=on  OutDataTypeStr=Inherit: Same as first input
  CoeffAct : Outport  InitialOutput=0
  wires:
  Gain1/1 -> Sum1/3
  Gain/1 -> Sum1/1
  Bus Selector/1 -> Aileron/1(Aileron)  "<da_rad>"
  Bus Selector1/1 -> Elevator/1(Elevator)  "<de_rad>"
  Bus Selector2/1 -> Rudder/1(Rudder)  "<dr_rad>"
  CMD/1 -> Bus Selector2/1, Bus Selector1/1, Bus Selector/1
  Sum1/1 -> CoeffAct/1
  Rudder/1(delCoeff) -> Gain1/1
  Aileron/1(delCoeff) -> Gain/1
  Elevator/1(delCoeff) -> Sum1/2

== system uavsimblockset/Cularis aerodynamics/Aerodynamics/Aerodynamic Coefficients Cularis/Body rate damping Increments ==
  pqr : Inport
  Va : Inport  Port=2
  Demux1 : Demux  Outputs=3
  Product3 : Product  Inputs=*/  SaturateOnIntegerOverflow=on  InputSameDT=on  OutDataTypeStr=Inherit: Same as first input
  Reference length c/2 : Gain  Gain=uavsim.CULARIS.c/2
  Reference span b/2 : Gain  Gain=uavsim.CULARIS.b/2
  "Reference span b/2 " : Gain  Gain=uavsim.CULARIS.b/2
  Sum1 : Sum  Inputs=+++  SaturateOnIntegerOverflow=on  InputSameDT=on  OutDataTypeStr=Inherit: Same as first input
  p : Subsystem
  q : Subsystem
  r : Subsystem
  CoeffRate : Outport  InitialOutput=0
  wires:
  pqr/1 -> Demux1/1
  Demux1/1 -> p/1(p)
  Demux1/2 -> q/1(q)
  Demux1/3 -> r/1(r)
  p/1(delCoeff) -> "Reference span b/2 "/1
  q/1(delCoeff) -> Reference length c/2/1
  r/1(delCoeff) -> Reference span b/2/1
  Product3/1 -> CoeffRate/1
  Sum1/1 -> Product3/1
  Va/1 -> Product3/2
  Reference span b/2/1 -> Sum1/3
  Reference length c/2/1 -> Sum1/2
  "Reference span b/2 "/1 -> Sum1/1

== system uavsimblockset/Cularis aerodynamics/Aerodynamics/Aerodynamic Coefficients Cularis/Datum Coefficients ==
  Alpha : Inport
  Beta : Inport  Port=2
  CD : Subsystem
  CL : Subsystem
  CY : Subsystem
  Cl : Subsystem
  Cm : Subsystem
  Cn : Subsystem
  Mux1 : Mux  Inputs=6
  CoeffDat : Outport  InitialOutput=0
  wires:
  Mux1/1 -> CoeffDat/1
  Alpha/1 -> CD/1(Alpha), CL/1(Alpha), Cm/1(Alpha)
  Beta/1 -> Cn/1(Beta), Cl/1(Beta), CY/1("Beta ")
  Cn/1(Cn) -> Mux1/6
  Cm/1(Cm) -> Mux1/5
  Cl/1("Cl ") -> Mux1/4
  CY/1(CY) -> Mux1/2
  CD/1(CD) -> Mux1/1
  CL/1(CL) -> Mux1/3

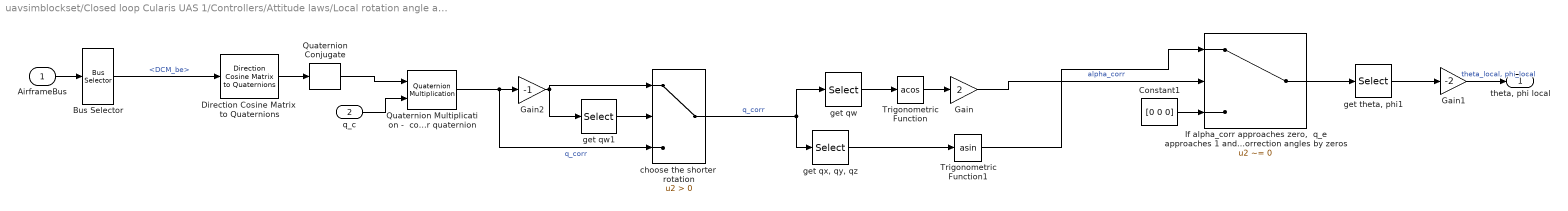
== system uavsimblockset/Closed loop Cularis UAS 1/Controllers/Attitude laws/Local rotation angle attitude  control/Compute local theta, phi, n_z ==
  AirframeBus : Inport  OutDataTypeStr=Bus: Airframe
  q_c : Inport  Port=2
  Bus Selector : BusSelector  OutputSignals=Kinematics.Attitude.DCM_be
  Constant1 : Constant  Value=[0 0 0]
  Direction Cosine Matrix  to Quaternions : aerolibtransform2/Direction Cosine Matrix  to Quaternions
  Gain : Gain  Gain=2
  Gain1 : Gain  Gain=-2
  Gain2 : Gain  Gain=-1
  "If alpha_corr approaches zero,  q_e approaches 1 and c goes to infinity.  In that case, just replace the computed  correction angles by zeros" : Switch  Criteria=u2 ~= 0
  Quaternion Conjugate : aerolibutil/Quaternion Conjugate
  Quaternion Multiplication -  compute error quaternion : aerolibutil/Quaternion Multiplication
  Trigonometric Function : Trigonometry  Operator=acos
  Trigonometric Function1 : Trigonometry  Operator=asin
  choose the shorter  rotation : Switch  Criteria=u2 > Threshold
  get qw : Selector  InputPortWidth=4  IndexOptions=Index vector (dialog)  Indices=1  OutputSizes=1
  get qw1 : Selector  InputPortWidth=4  IndexOptions=Index vector (dialog)  Indices=1  OutputSizes=1
  "get qx, qy, qz" : Selector  InputPortWidth=4  IndexOptions=Index vector (dialog)  Indices=2:4  OutputSizes=1
  "get theta, phi1" : Selector  InputPortWidth=3  IndexOptions=Index vector (dialog)  Indices=[2 1]  OutputSizes=1
  "theta, phi local" : Outport
  wires:
  Direction Cosine Matrix  to Quaternions/1 -> Quaternion Conjugate/1
  get qw1/1 -> choose the shorter  rotation/2
  Gain2/1 -> get qw1/1, choose the shorter  rotation/1
  Quaternion Multiplication -  compute error quaternion/1 -> Gain2/1, choose the shorter  rotation/3  "q_corr"
  Gain1/1 -> "theta, phi local"/1  "theta_local, phi_local"
  Quaternion Conjugate/1 -> Quaternion Multiplication -  compute error quaternion/1
  "get theta, phi1"/1 -> Gain1/1
  "If alpha_corr approaches zero,  q_e approaches 1 and c goes to infinity.  In that case, just replace the computed  correction angles by zeros"/1 -> "get theta, phi1"/1
  Constant1/1 -> "If alpha_corr approaches zero,  q_e approaches 1 and c goes to infinity.  In that case, just replace the computed  correction angles by zeros"/3
  Trigonometric Function1/1 -> "If alpha_corr approaches zero,  q_e approaches 1 and c goes to infinity.  In that case, just replace the computed  correction angles by zeros"/1
  "get qx, qy, qz"/1 -> Trigonometric Function1/1
  Gain/1 -> "If alpha_corr approaches zero,  q_e approaches 1 and c goes to infinity.  In that case, just replace the computed  correction angles by zeros"/2  "alpha_corr"
  Trigonometric Function/1 -> Gain/1
  get qw/1 -> Trigonometric Function/1
  choose the shorter  rotation/1 -> "get qx, qy, qz"/1, get qw/1  "q_corr"
  q_c/1 -> Quaternion Multiplication -  compute error quaternion/2
  Bus Selector/1 -> Direction Cosine Matrix  to Quaternions/1  "<DCM_be>"
  AirframeBus/1 -> Bus Selector/1

== system uavsimblockset/Closed loop Cularis UAS 1/Controllers/Attitude laws/Local rotation angle attitude  control/LQR pitch ==
  q : Inport
  theta : Inport  Port=2
  theta_c : Inport  Port=3
  Add1 : Sum  Inputs=-+
  Integrator1 : Integrator
  Mux2 : Mux  Inputs=3
  lquadr gain : Gain  Gain=uavsim.ap.control.lquadr.pitch.K  Multiplication=Matrix(K*u)
  de : Outport
  wires:
  lquadr gain/1 -> de/1  "de"
  Integrator1/1 -> Mux2/3
  Mux2/1 -> lquadr gain/1
  theta/1 -> Add1/2
  theta_c/1 -> Add1/1
  Add1/1 -> Integrator1/1, Mux2/1  "e"
  q/1 -> Mux2/2

== system uavsimblockset/Closed loop Cularis UAS 1/Controllers/Attitude laws/Local rotation angle attitude  control/LQR roll ==
  phi : Inport
  phi_c : Inport  Port=2
  p : Inport  Port=3
  r : Inport  Port=4
  Add1 : Sum  Inputs=-+
  Demux : Demux  Outputs=2
  Integrator : Integrator
  Mux2 : Mux
  lquadr gain : Gain  Gain=uavsim.ap.control.lquadr.minimal.K  Multiplication=Matrix(K*u)
  da : Outport
  dr : Outport  Port=2
  wires:
  Demux/2 -> dr/1
  lquadr gain/1 -> Demux/1
  r/1 -> Mux2/3
  Integrator/1 -> Mux2/4
  Mux2/1 -> lquadr gain/1
  phi/1 -> Add1/2
  phi_c/1 -> Add1/1
  Add1/1 -> Integrator/1, Mux2/1  "e"
  Demux/1 -> da/1
  p/1 -> Mux2/2

== system uavsimblockset/Cularis aerodynamics/Aerodynamics/Aerodynamic Coefficients Cularis/Actuator Increments/Aileron ==
  Aileron : Inport
  CY_da : Gain  Gain=uavsim.CULARIS.CY_da
  Cl_da : Gain  Gain=uavsim.CULARIS.Cl_da
  Cn_da : Gain  Gain=uavsim.CULARIS.Cn_da
  Constant : Constant  Value=0
  Constant1 : Constant  Value=0
  Constant2 : Constant  Value=0
  Mux1 : Mux  Inputs=6
  delCoeff : Outport
  wires:
  Constant2/1 -> Mux1/5
  Constant1/1 -> Mux1/3
  Aileron/1 -> Cl_da/1, Cn_da/1, CY_da/1
  Constant/1 -> Mux1/1
  Mux1/1 -> delCoeff/1
  CY_da/1 -> Mux1/2
  Cl_da/1 -> Mux1/4
  Cn_da/1 -> Mux1/6

== system uavsimblockset/Cularis aerodynamics/Aerodynamics/Aerodynamic Coefficients Cularis/Actuator Increments/Elevator ==
  Elevator : Inport
  CD_de : Gain  Gain=uavsim.CULARIS.CD_de
  CL_de : Gain  Gain=uavsim.CULARIS.CL_de
  Cm_de : Gain  Gain=uavsim.CULARIS.Cm_de
  Constant : Constant  Value=0
  Constant1 : Constant  Value=0
  Constant2 : Constant  Value=0
  Mux1 : Mux  Inputs=6
  delCoeff : Outport
  wires:
  Constant2/1 -> Mux1/6
  Constant1/1 -> Mux1/4
  Elevator/1 -> CL_de/1, CD_de/1, Cm_de/1
  CD_de/1 -> Mux1/1
  Mux1/1 -> delCoeff/1
  CL_de/1 -> Mux1/3
  Cm_de/1 -> Mux1/5
  Constant/1 -> Mux1/2

== system uavsimblockset/Cularis aerodynamics/Aerodynamics/Aerodynamic Coefficients Cularis/Actuator Increments/Rudder ==
  Rudder : Inport
  CY_dr : Gain  Gain=uavsim.CULARIS.CY_dr
  Cl_dr : Gain  Gain=uavsim.CULARIS.Cl_dr
  Cn_dr : Gain  Gain=uavsim.CULARIS.Cn_dr
  Constant : Constant  Value=0
  Constant1 : Constant  Value=0
  Constant2 : Constant  Value=0
  Mux1 : Mux  Inputs=6
  delCoeff : Outport
  wires:
  Constant2/1 -> Mux1/5
  Constant1/1 -> Mux1/3
  Rudder/1 -> Cl_dr/1, Cn_dr/1, CY_dr/1
  Mux1/1 -> delCoeff/1
  CY_dr/1 -> Mux1/2
  Cl_dr/1 -> Mux1/4
  Cn_dr/1 -> Mux1/6
  Constant/1 -> Mux1/1

== system uavsimblockset/Cularis aerodynamics/Aerodynamics/Aerodynamic Coefficients Cularis/Body rate damping Increments/p ==
  p : Inport
  CY_p : Gain  Gain=uavsim.CULARIS.CY_p
  Cl_p : Gain  Gain=uavsim.CULARIS.Cl_p
  Cn_p : Gain  Gain=uavsim.CULARIS.Cn_p
  Constant1 : Constant  Value=0
  Constant2 : Constant  Value=0
  Constant3 : Constant  Value=0
  Gain : Gain
  Gain1 : Gain
  Mux1 : Mux  Inputs=6
  delCoeff : Outport
  wires:
  Gain1/1 -> Mux1/6
  Gain/1 -> Mux1/4
  Constant3/1 -> Mux1/5
  Constant2/1 -> Mux1/3
  Mux1/1 -> delCoeff/1
  Cl_p/1 -> Gain/1
  Cn_p/1 -> Gain1/1
  Constant1/1 -> Mux1/1
  CY_p/1 -> Mux1/2
  p/1 -> CY_p/1, Cl_p/1, Cn_p/1

== system uavsimblockset/Cularis aerodynamics/Aerodynamics/Aerodynamic Coefficients Cularis/Body rate damping Increments/q ==
  q : Inport
  CD_q : Gain  Gain=uavsim.CULARIS.CD_q
  CL_q : Gain  Gain=uavsim.CULARIS.CL_q
  Cm_q : Gain  Gain=uavsim.CULARIS.Cm_q
  Constant1 : Constant  Value=0
  Constant2 : Constant  Value=0
  Constant3 : Constant  Value=0
  Mux1 : Mux  Inputs=6
  delCoeff : Outport
  wires:
  Constant3/1 -> Mux1/6
  Constant2/1 -> Mux1/4
  Mux1/1 -> delCoeff/1
  q/1 -> CD_q/1, CL_q/1, Cm_q/1
  Constant1/1 -> Mux1/2
  CD_q/1 -> Mux1/1
  CL_q/1 -> Mux1/3
  Cm_q/1 -> Mux1/5

== system uavsimblockset/Cularis aerodynamics/Aerodynamics/Aerodynamic Coefficients Cularis/Body rate damping Increments/r ==
  r : Inport
  CY_r : Gain  Gain=uavsim.CULARIS.CY_r
  Cl_r : Gain  Gain=uavsim.CULARIS.Cl_r
  Cn_r : Gain  Gain=uavsim.CULARIS.Cn_r
  Constant1 : Constant  Value=0
  Constant2 : Constant  Value=0
  Constant3 : Constant  Value=0
  Mux1 : Mux  Inputs=6
  delCoeff : Outport
  wires:
  Constant3/1 -> Mux1/5
  Constant2/1 -> Mux1/3
  Mux1/1 -> delCoeff/1
  r/1 -> CY_r/1, Cl_r/1, Cn_r/1
  Constant1/1 -> Mux1/1
  CY_r/1 -> Mux1/2
  Cl_r/1 -> Mux1/4
  Cn_r/1 -> Mux1/6

== system uavsimblockset/Cularis aerodynamics/Aerodynamics/Aerodynamic Coefficients Cularis/Datum Coefficients/CD ==
  Alpha : Inport
  CD_0 : Constant  Value=uavsim.CULARIS.CD_0
  CL_0 : Constant  Value=uavsim.CULARIS.CL_0
  CL_alpha : Gain  Gain=uavsim.CULARIS.CL_alpha
  Product : Product  RndMeth=Zero
  Sum1 : Sum  Inputs=|++
  Sum2 : Sum  Inputs=|++
  sec. order lift contribution : Gain  Gain=1/(pi*uavsim.CULARIS.oswald*uavsim.CULARIS.AR )
  CD : Outport
  wires:
  CL_0/1 -> Sum2/1
  Sum2/1 -> Product/2, Product/1
  Product/1 -> sec. order lift contribution/1
  sec. order lift contribution/1 -> Sum1/1
  CD_0/1 -> Sum1/2
  Sum1/1 -> CD/1
  Alpha/1 -> CL_alpha/1
  CL_alpha/1 -> Sum2/2
